simulink subsystem "thrust_mode"  (R2021a)
settings: Solver=VariableStepAuto  StartTime=0.0  StopTime=10.0  RelTol=1e-3
settings Model: Creator=EpEp  LastModifiedBy=EpEp

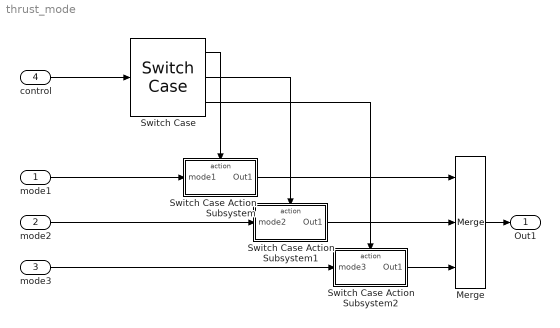
== system thrust_mode ==
  mode1 : Inport
  mode2 : Inport  Port=2
  mode3 : Inport  Port=3
  control : Inport  Port=4
  Merge : Merge  Inputs=3
  Switch Case : SwitchCase  CaseConditions={1,2,3}  ShowDefaultCase=off
  Switch Case Action Subsystem : Subsystem  TreatAsAtomicUnit=on
  Switch Case Action Subsystem1 : Subsystem  TreatAsAtomicUnit=on
  Switch Case Action Subsystem2 : Subsystem  TreatAsAtomicUnit=on
  Out1 : Outport
  wires:
  Switch Case/1 -> Switch Case Action Subsystem/Action
  Switch Case/2 -> Switch Case Action Subsystem1/Action
  Switch Case/3 -> Switch Case Action Subsystem2/Action
  control/1 -> Switch Case/1
  mode1/1 -> Switch Case Action Subsystem/1(mode1)
  mode2/1 -> Switch Case Action Subsystem1/1(mode2)
  mode3/1 -> Switch Case Action Subsystem2/1(mode3)
  Merge/1 -> Out1/1
  Switch Case Action Subsystem2/1(Out1) -> Merge/3
  Switch Case Action Subsystem1/1(Out1) -> Merge/2
  Switch Case Action Subsystem/1(Out1) -> Merge/1

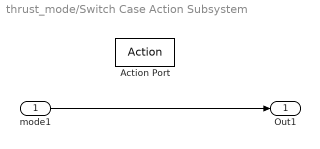
== system thrust_mode/Switch Case Action Subsystem ==
  mode1 : Inport
  Action Port : ActionPort
  Out1 : Outport
  wires:
  mode1/1 -> Out1/1

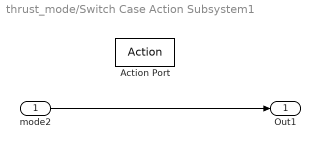
== system thrust_mode/Switch Case Action Subsystem1 ==
  mode2 : Inport
  Action Port : ActionPort
  Out1 : Outport
  wires:
  mode2/1 -> Out1/1

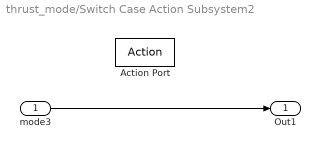
== system thrust_mode/Switch Case Action Subsystem2 ==
  mode3 : Inport
  Action Port : ActionPort
  Out1 : Outport
  wires:
  mode3/1 -> Out1/1
